simulink model "space_state"  (R2024a)
settings: Solver=VariableStepAuto  StartTime=0.0  StopTime=10.0  RelTol=1e-3
values from neighbouring files (symbols this model uses):
  f = (1-phi_m)/gamma_m    [electrical_mechanical_parameters.m]
  J = -(f*h)/log(phi_m)    [electrical_mechanical_parameters.m]
  Ka = Kg    [electrical_mechanical_parameters.m]
  Kg = Kt*(w'*e)/(w'*w)    [computing_Kg.m]    (also in electrical_mechanical_parameters.m = Kg)
  La = -(Ra*h)/log(phi_e)    [electrical_mechanical_parameters.m]
  Ra = (1-phi_e)/gamma_e    [electrical_mechanical_parameters.m]
undefined symbols (not defined in the file or in its folder): Kt
settings Model: Creator=Guilherme  LastModifiedBy=Guilherme

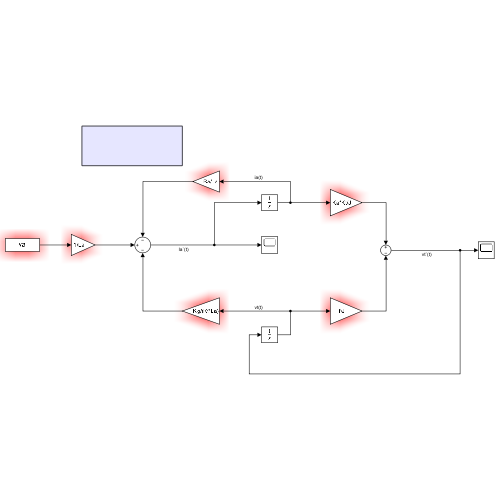
[thumbnail: Simulink's stored preview of the top-level diagram]
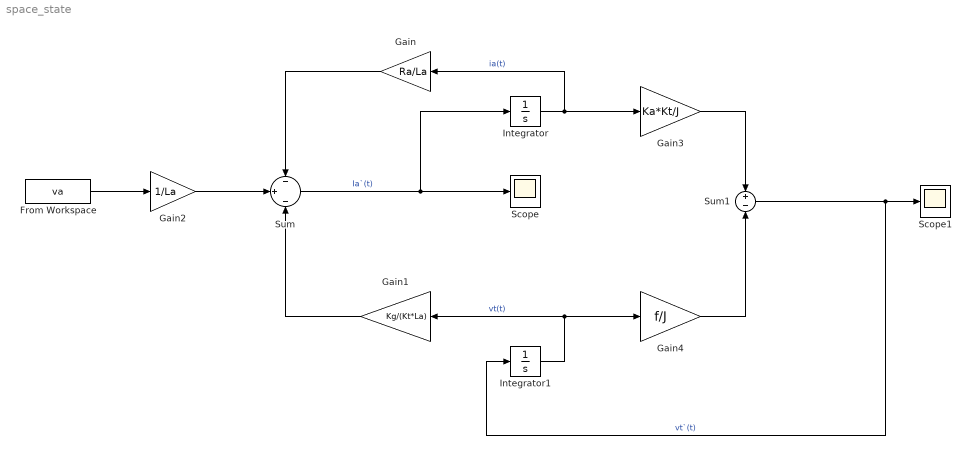
== system space_state ==
  From Workspace : FromWorkspace  VariableName=va
  Gain : Gain  Gain=Ra/La
  Gain1 : Gain  Gain=Kg/(Kt*La)
  Gain2 : Gain  Gain=1/La
  Gain3 : Gain  Gain=Ka*Kt/J
  Gain4 : Gain  Gain=f/J
  Integrator : Integrator
  Integrator1 : Integrator
  Scope : Scope
  Scope1 : Scope
  Sum : Sum  Inputs=-|+|-
  Sum1 : Sum  Inputs=+|-
  wires:
  Integrator/1 -> Gain3/1, Gain/1  "ia(t)"
  Integrator1/1 -> Gain4/1, Gain1/1  "vt(t)"
  Gain/1 -> Sum/1
  Gain1/1 -> Sum/3
  Gain2/1 -> Sum/2
  Sum/1 -> Integrator/1, Scope/1  "Ia`(t)"
  Sum1/1 -> Integrator1/1, Scope1/1  "vt`(t)"
  Gain4/1 -> Sum1/2
  Gain3/1 -> Sum1/1
  From Workspace/1 -> Gain2/1
